simulink model "W04_3_heading"  (R2024b)
settings: Solver=ode4  StartTime=0.0  StopTime=inf  FixedStep=0.05  RelTol=1e-3
values from neighbouring files (symbols this model uses):
  animate = 1    [W04_setup.m]
  head_open = 0    [W04_setup.m]
  Kd_psi = 400    [W04_setup.m]
  Ki_psi = 0    [W04_setup.m]
  Kp_psi = 800    [W04_setup.m]
  N_max = 500    [W04_setup.m]
  N_open = 300    [W04_setup.m]
  port_eff = 1.0    (= 1)    [W04_setup.m]
  psi_ref_deg = 45    [W04_setup.m]
  use_ssa = 1    [W04_setup.m]
  X_head = 300    [W04_setup.m]
libraries: ros2lib x5
settings Model: Creator=admin  LastModifiedBy=admin

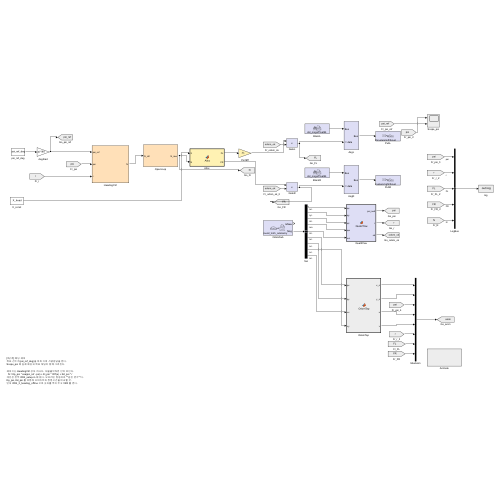
[thumbnail: Simulink's stored preview of the top-level diagram]
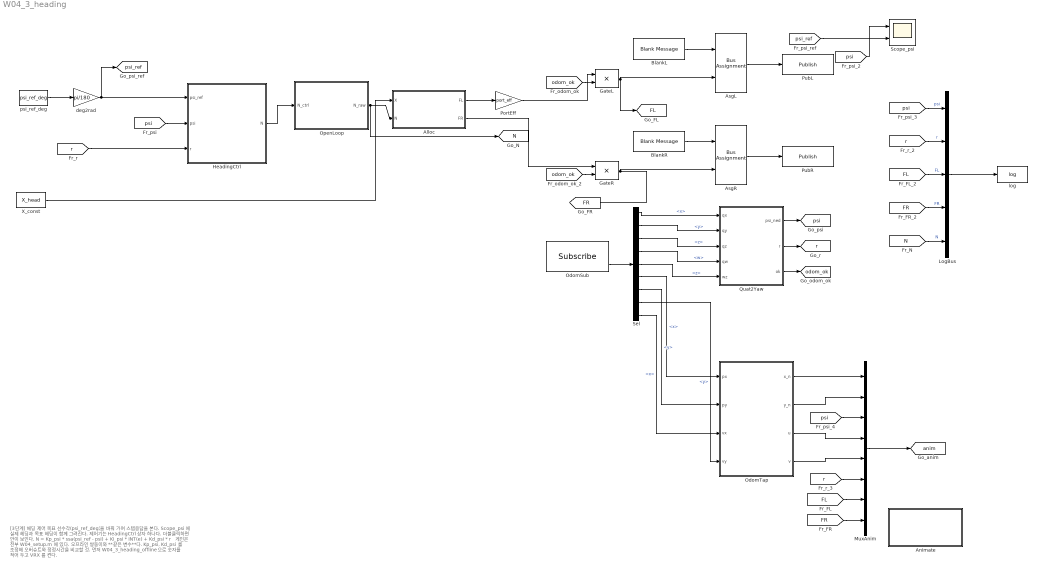
== system W04_3_heading ==
  note: [3단계] 헤딩 제어
      | 목표 선수각(psi_ref_deg)을 바꿔 가며 스텝응답을 본다.
      | Scope_psi 에 실제 헤딩과 목표 헤딩이 함께 그려진다.
      |
      | 제어기는 HeadingCtrl 상자 하나다. 더블클릭하면 안이 보인다.
      |   N = Kp_psi * ssa(psi_ref - psi) + Ki_psi * INT(e) + Kd_psi * r
      | 게인은 전부 W04_setup.m 에 있다. 오프라인 쌍둥이와 **같은 변수**다.
      | Kp_psi, Kd_psi 를 조정해 오버슈트와 정정시간을 비교할 것.
      | 먼저 W04_3_heading_offline 으로 숫자를 적어 두고 VRX 를 켠다.
  Alloc : MATLAB Function  TreatAsAtomicUnit=on
  Animate : Subsystem
  AsgL : BusAssignment  AssignedSignals=data
  AsgR : BusAssignment  AssignedSignals=data
  BlankL : ros2lib/Blank Message  messageClass=Message  entityType=std_msgs/Float64  messageType=std_msgs/Float64  SampleTime=0.05
  BlankR : ros2lib/Blank Message  messageClass=Message  entityType=std_msgs/Float64  messageType=std_msgs/Float64  SampleTime=0.05
  GateL : Product
  GateR : Product
  HeadingCtrl : Subsystem
  LogBus : BusCreator  Inputs=5
  MuxAnim : Mux  Inputs=8
  OdomSub : ros2lib/Subscribe  topicSource=Specify your own  topic=/wamv/sensors/position/ground_truth_odometry  messageType=nav_msgs/Odometry  sampleTime=0.05  QOSHistory=Keep last  QOSDepth=1  QOSReliability=Reliable  QOSDurability=Volatile  QOSDeadline=Inf  QOSLifespan=Inf  QOSLiveliness=Automatic  QOSLeaseDuration=Inf  QOSAvoidROSNamespaceConventions=off
  OdomTap : MATLAB Function  TreatAsAtomicUnit=on
  OpenLoop : Subsystem
  PortEff : Gain  Gain=port_eff
  PubL : ros2lib/Publish  topicSource=Specify your own  topic=/wamv/thrusters/left/thrust  messageType=std_msgs/Float64  QOSHistory=Keep last  QOSDepth=1  QOSReliability=Reliable  QOSDurability=Volatile  QOSDeadline=Inf  QOSLifespan=Inf  QOSLiveliness=Automatic  QOSLeaseDuration=Inf  QOSAvoidROSNamespaceConventions=off
  PubR : ros2lib/Publish  topicSource=Specify your own  topic=/wamv/thrusters/right/thrust  messageType=std_msgs/Float64  QOSHistory=Keep last  QOSDepth=1  QOSReliability=Reliable  QOSDurability=Volatile  QOSDeadline=Inf  QOSLifespan=Inf  QOSLiveliness=Automatic  QOSLeaseDuration=Inf  QOSAvoidROSNamespaceConventions=off
  Quat2Yaw : MATLAB Function  TreatAsAtomicUnit=on
  Scope_psi : Scope  NumInputPorts=2
  Sel : BusSelector  OutputSignals=pose.pose.orientation.x,pose.pose.orientation.y,pose.pose.orientation.z,pose.pose.orientation.w,twist.twist.angular.z,pose.pose.position.x,pose.pose.position.y,twist.twist.linear.y,twist.twist.linear.x
  X_const : Constant  Value=X_head
  deg2rad : Gain  Gain=pi/180
  log : ToWorkspace  VariableName=log  SaveFormat=Timeseries  SampleTime=0.05
  psi_ref_deg : Constant  Value=psi_ref_deg
  tag scope: FL=global, FR=global, N=global, anim=global, odom_ok=global, psi=global, psi_ref=global, r=global
  wires:
  OdomSub/2 -> Sel/1
  Sel/2 -> Quat2Yaw/2(qy)  "<y>"
  Sel/3 -> Quat2Yaw/3(qz)  "<z>"
  Sel/4 -> Quat2Yaw/4(qw)  "<w>"
  Sel/5 -> Quat2Yaw/5(wz)  "<z>"
  Quat2Yaw/1(psi_ned) -> [psi]
  Quat2Yaw/2(r) -> [r]
  Quat2Yaw/3(ok) -> [odom_ok]
  Sel/6 -> OdomTap/1(px)  "<x>"
  Sel/7 -> OdomTap/2(py)  "<y>"
  Sel/9 -> OdomTap/3(vx)  "<x>"
  Sel/8 -> OdomTap/4(vy)  "<y>"
  OdomTap/1(x_n) -> MuxAnim/1
  OdomTap/2(y_n) -> MuxAnim/2
  OdomTap/3(u) -> MuxAnim/4
  OdomTap/4(v) -> MuxAnim/5
  [FL] -> MuxAnim/7
  [FR] -> MuxAnim/8
  MuxAnim/1 -> [anim]
  HeadingCtrl/1(N) -> OpenLoop/1(N_ctrl)
  OpenLoop/1(N_raw) -> Alloc/2(N), [N]
  psi_ref_deg/1 -> deg2rad/1
  deg2rad/1 -> HeadingCtrl/1(psi_ref), [psi_ref]
  [psi] -> HeadingCtrl/2(psi)
  [r] -> HeadingCtrl/3(r)
  Alloc/1(FL) -> PortEff/1
  BlankL/1 -> AsgL/1
  AsgL/1 -> PubL/1
  BlankR/1 -> AsgR/1
  AsgR/1 -> PubR/1
  PortEff/1 -> GateL/1
  [odom_ok] -> GateL/2
  GateL/1 -> AsgL/2, [FL]
  Alloc/2(FR) -> GateR/1
  [odom_ok] -> GateR/2
  [psi] -> Scope_psi/1
  [psi_ref] -> Scope_psi/2
  [psi] -> LogBus/1  "psi"
  [r] -> LogBus/2  "r"
  [FL] -> LogBus/3  "FL"
  [FR] -> LogBus/4  "FR"
  [N] -> LogBus/5  "N"
  LogBus/1 -> log/1
  [r] -> MuxAnim/6
  [psi] -> MuxAnim/3
  X_const/1 -> Alloc/1(X)
  Sel/1 -> Quat2Yaw/1(qx)  "<x>"
  GateR/1 -> AsgR/2, [FR]

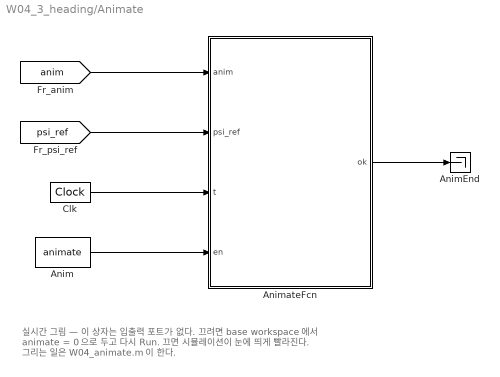
== system W04_3_heading/Animate ==
  note: 실시간 그림 — 이 상자는 입출력 포트가 없다.
      | 끄려면 base workspace 에서  animate = 0  으로 두고 다시 Run.
      | 끄면 시뮬레이션이 눈에 띄게 빨라진다.
      | 그리는 일은 W04_animate.m 이 한다.
  Anim : Constant  Value=animate
  AnimEnd : Terminator
  AnimateFcn : MATLAB Function  TreatAsAtomicUnit=on
  Clk : DigitalClock  SampleTime=0.05
  wires:
  [anim] -> AnimateFcn/1(anim)
  [psi_ref] -> AnimateFcn/2(psi_ref)
  Clk/1 -> AnimateFcn/3(t)
  Anim/1 -> AnimateFcn/4(en)
  AnimateFcn/1(ok) -> AnimEnd/1

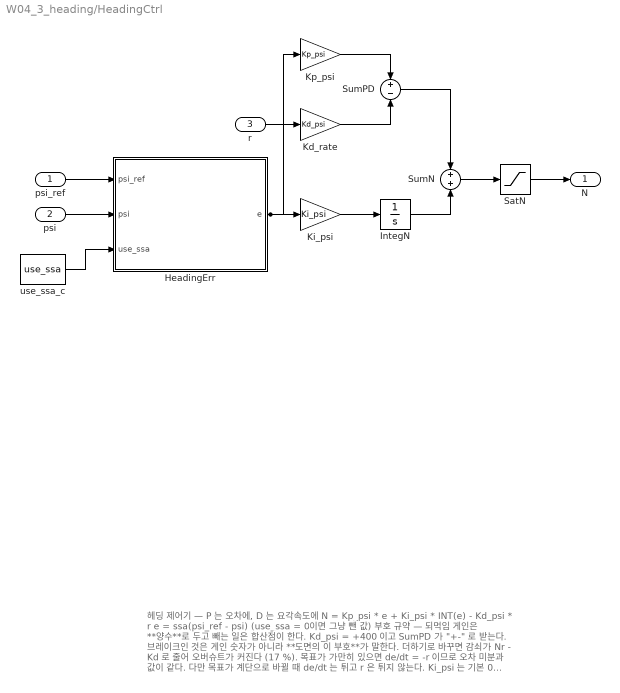
== system W04_3_heading/HeadingCtrl ==
  note: 헤딩 제어기 — P 는 오차에, D 는 요각속도에
      |
      |     N = Kp_psi * e  +  Ki_psi * INT(e)  -  Kd_psi * r
      |     e = ssa(psi_ref - psi)   (use_ssa = 0 이면 그냥 뺀 값)
      |
      | 부호 규약 — 되먹임 게인은 **양수**로 두고 빼는 일은 합산점이 한다.
      | Kd_psi = +400 이고 SumPD 가 "+-" 로 받는다. 브레이크인 것은 게인
      | 숫자가 아니라 **도면의 이 부호**가 말한다.
      | 더하기로 바꾸면 감쇠가 Nr - Kd 로 줄어 오버슈트가 커진다 (17 %).
      |
      | 목표가 가만히 있으면 de/dt = -r 이므로 오차 미분과 값이 같다.
      | 다만 목표가 계단으로 바뀔 때 de/dt 는 튀고 r 은 튀지 않는다.
      |
      | Ki_psi 는 기본 0 이다. 한쪽 추진기가 약할 때(port_eff < 1)
      | PD 가 남기는 정상상태 오차를 없애는 자리다 (2-10 절 실습에서 켠다).
      | IntegN 은 **연속** 적분기이고 +-N_max 포화가 걸려 있다
      | (clamping 안티와인드업). 모델 솔버는 고정스텝 ode4 다.
      |
      | SatN 의 +-N_max = 500 N m 는 임의의 수가 아니다. 추진기만으로 낼 수
      | 있는 물리 한계가 2*b_half*F_max = 2*1.027135*250 = 513.57 N m 이고,
      | 500 은 그 97.4 % 다. 전진 추력 X 를 함께 쓰면 2*b_half*(F_max - X/2)
      | 로 줄어, X_head = 300 N 에서는 205.4 N m 가 진짜 한계다 (2-5 절 유도 5).
      |
      | 값은 전부 W04_setup.m — Kp_psi = 800, Kd_psi = +400.
      | 근거는 4주차 극배치 절과 W04_pole_place.m.
  psi_ref : Inport
  psi : Inport  Port=2
  r : Inport  Port=3
  HeadingErr : MATLAB Function  TreatAsAtomicUnit=on
  IntegN : Integrator  LimitOutput=on  UpperSaturationLimit=N_max  LowerSaturationLimit=-N_max
  Kd_rate : Gain  Gain=Kd_psi
  Ki_psi : Gain  Gain=Ki_psi
  Kp_psi : Gain  Gain=Kp_psi
  SatN : Saturate  UpperLimit=N_max  LowerLimit=-N_max
  SumN : Sum
  SumPD : Sum  Inputs=+-
  use_ssa_c : Constant  Value=use_ssa
  N : Outport
  wires:
  psi/1 -> HeadingErr/2(psi)
  psi_ref/1 -> HeadingErr/1(psi_ref)
  HeadingErr/1(e) -> Kp_psi/1, Ki_psi/1
  use_ssa_c/1 -> HeadingErr/3(use_ssa)
  Kp_psi/1 -> SumPD/1
  r/1 -> Kd_rate/1
  Kd_rate/1 -> SumPD/2
  Ki_psi/1 -> IntegN/1
  SumPD/1 -> SumN/1
  IntegN/1 -> SumN/2
  SumN/1 -> SatN/1
  SatN/1 -> N/1

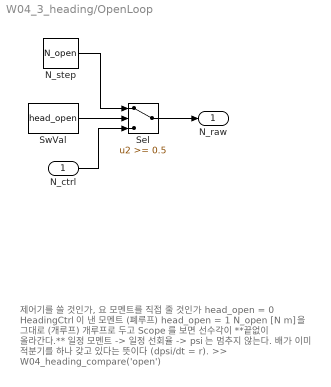
== system W04_3_heading/OpenLoop ==
  note: 제어기를 쓸 것인가, 요 모멘트를 직접 줄 것인가
      |
      |   head_open = 0   HeadingCtrl 이 낸 모멘트 (폐루프)
      |   head_open = 1   N_open [N m] 을 그대로 (개루프)
      |
      | 개루프로 두고 Scope 를 보면 선수각이 **끝없이 올라간다.**
      | 일정 모멘트 -> 일정 선회율 -> psi 는 멈추지 않는다.
      | 배가 이미 적분기를 하나 갖고 있다는 뜻이다 (dpsi/dt = r).
      |
      |   >> W04_heading_compare('open')
  N_ctrl : Inport
  N_step : Constant  Value=N_open
  Sel : Switch  Threshold=0.5  SaturateOnIntegerOverflow=off  InputSameDT=off
  SwVal : Constant  Value=head_open
  N_raw : Outport
  wires:
  Sel/1 -> N_raw/1
  N_step/1 -> Sel/1
  SwVal/1 -> Sel/2
  N_ctrl/1 -> Sel/3

== matlab function W04_3_heading/OdomTap ==
  data: px input; x_n output; py input; vx input; vy input; y_n output; u output; v output
function [x_n, y_n, u, v] = OdomTap(px, py, vx, vy)
%#codegen
% Ground truth odometry -> the numbers the live plot draws.
% Display only: nothing here feeds the controller.
x_n = py;      % ENU y is north
y_n = px;      % ENU x is east
u   =  vx;     % surge is the same in FLU and NED body axes
v   = -vy;     % FLU +y is port, NED +y is starboard

== matlab function W04_3_heading/Quat2Yaw ==
  data: qx input; psi_ned output; qy input; qz input; qw input; wz input; r output; ok output
function [psi_ned, r, ok] = Quat2Yaw(qx, qy, qz, qw, wz)
%#codegen
% ROS quaternion (ENU body) -> NED heading [rad] and yaw rate [rad/s]
yaw_enu = atan2(2*(qw*qz + qx*qy), 1 - 2*(qy*qy + qz*qz));
psi = pi/2 - yaw_enu;
psi_ned = atan2(sin(psi), cos(psi));   % wrap to [-pi, pi]

% psi_ned = pi/2 - yaw_enu  ->  d(psi_ned)/dt = -d(yaw_enu)/dt.
% ENU is z-up and NED is z-down, so the turn direction flips.
r = -wz;

% ok = 0 holds the thrusters at 0 (addFirstMsgGate). Two reasons:
%  1) Before the first odometry arrives the Subscribe block outputs an all-zero bus.
%     A zero quaternion reads as exactly 90 deg.
%  2) Simulink stalls for up to a few wall-clock seconds in its first steps while
%     Gazebo keeps running on the first thrust command. The boat turned 9 to 55 deg
%     before the model resumed (2026-09-24). So wait 1 s (20 samples) after the first
%     valid message, then start the step from a boat that is still at rest.
persistent n
if isempty(n), n = 0; end
valid = qx ~= 0 || qy ~= 0 || qz ~= 0 || qw ~= 0;
if valid, n = n + 1; end
ok = double(valid && n > 20);

== matlab function W04_3_heading/HeadingCtrl/HeadingErr ==
  data: psi_ref input; e output; psi input; use_ssa input
function e = HeadingErr(psi_ref, psi, use_ssa)
%#codegen
% Heading error [rad].
d = psi_ref - psi;
if use_ssa >= 0.5
    % ssa : shortest signed angle, wrapped to (-pi, pi]
    e = atan2(sin(d), cos(d));
else
    % no wrap : 170 deg -> -170 deg becomes -340 deg, not +20 deg
    e = d;
end

== matlab function W04_3_heading/Alloc ==
  data: X input; FL output; N input; FR output
function [FL, FR] = Alloc(X, N)
%#codegen
% Differential thrust allocation for the 2-thruster WAM-V
%   X : surge force  [N]
%   N : yaw moment   [N*m], positive turns to starboard
B_half = 1.027135;      % half distance between thrusters [m]
Fmax   = 250;           % thrust limit per thruster [N]
FL = X/2 + N/(2*B_half);
FR = X/2 - N/(2*B_half);
FL = max(min(FL, Fmax), -Fmax);
FR = max(min(FR, Fmax), -Fmax);

== matlab function W04_3_heading/Animate/AnimateFcn ==
  data: anim input; ok output; psi_ref input; t input; en input
function ok = AnimateFcn(anim, psi_ref, t, en)
%#codegen
% 실시간 그림. MATLAB Function 블록은 그림을 그리지 못하므로 그리는 함수를
% extrinsic 으로 선언한다 — 코드를 만들지 않고 평범한 MATLAB 을 부른다.
% en = base workspace 의 animate (0 이면 그리지 않는다).
%
% anim 은 Mux 로 묶어 온 여덟 신호다 (빌더의 animBundle 과 같은 순서).
%   1 x_n   2 y_n   3 psi   4 u   5 v   6 r   7 FL   8 FR
coder.extrinsic('W04_animate');
ok = 1;
if en > 0.5
    W04_animate(anim(1), anim(2), anim(3), anim(4), anim(5), anim(6), anim(7), anim(8), NaN, psi_ref, t);
end
